simulink model "hw3_1b_Stimulation"  (R2013a)
settings: Solver=ode45  StartTime=0.0  StopTime=1  MaxStep=0.01  RelTol=1e-3
libraries: simulink x1
settings Model: Creator=benshih  LastModifiedBy=benshih

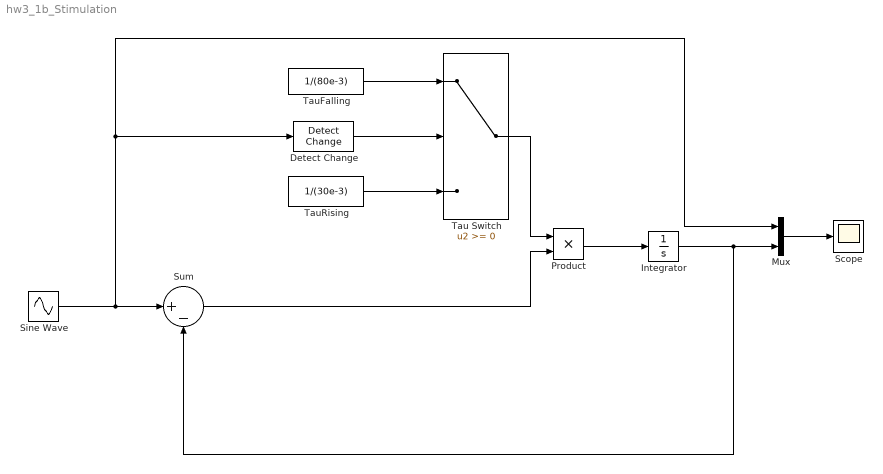
== system hw3_1b_Stimulation ==
  Detect Change : simulink/Logic and Bit Operations/Detect Change  vinit=0  InputProcessing=Inherited  OutDataTypeStr=uint8
  Integrator : Integrator
  Mux : Mux  Inputs=2
  Product : Product
  Scope : Scope
  Sine Wave : Sin  Amplitude=1/2  Bias=1/2  Frequency=2*pi*5  SampleTime=0
  Sum : Sum  Inputs=|+-
  Tau Switch : Switch
  TauFalling : Constant  Value=1/(80e-3)
  TauRising : Constant  Value=1/(30e-3)
  wires:
  Sine Wave/1 -> Mux/1, Detect Change/1, Sum/1
  Integrator/1 -> Mux/2, Sum/2
  TauFalling/1 -> Tau Switch/1
  TauRising/1 -> Tau Switch/3
  Detect Change/1 -> Tau Switch/2
  Sum/1 -> Product/2
  Tau Switch/1 -> Product/1
  Product/1 -> Integrator/1
  Mux/1 -> Scope/1
